simulink model "Inverse_Stewartplatform"  (R2024a)
settings: Solver=VariableStepAuto  StartTime=0.0  StopTime=0  RelTol=1e-3
settings Model: Creator=Challa  LastModifiedBy=Challa

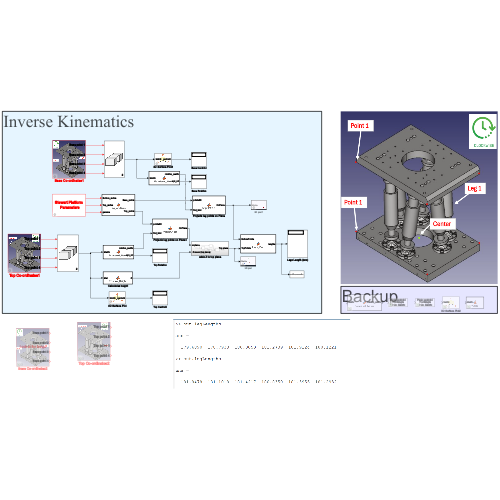
[thumbnail: Simulink's stored preview of the top-level diagram]
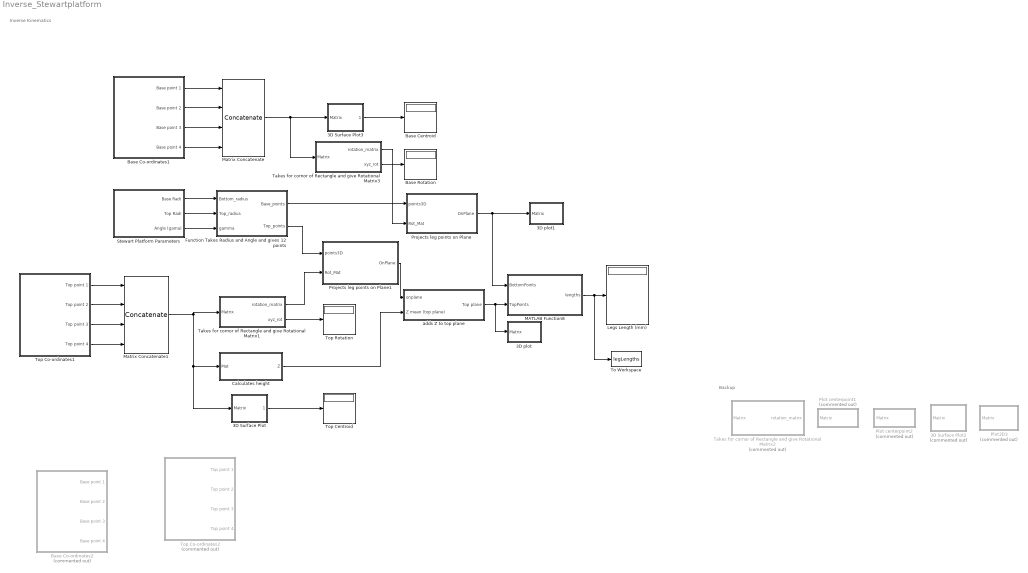
== system Inverse_Stewartplatform ==
  note: Backup
  note: Inverse Kinematics
  3D Surface Plot : Subsystem  mask(3D Surface Plot){color2='r'}
      mask prompts: color2 "color"
      mask help:
      | Input: 3xN matrix
      | output: 3D Surface Plot
      | Color: Changable by giving input
      | Finds Centerpoint and plots.
      mask Help:
      | Input: 3xN matrix
      | output: 3D Surface Plot
      | Color: Changable by giving input
      | Finds Centerpoint and plots.
      mask Display: image('XYZ2.png');
  3D Surface Plot2 : Subsystem  Commented=on  mask(3D Surface Plot){color2='b'}
      mask prompts: color2 "color"
      mask help:
      | Input: 3xN matrix
      | output: 3D Surface Plot
      | Color: Changable by giving input
      | Finds Centerpoint and plots.
      mask Help:
      | Input: 3xN matrix
      | output: 3D Surface Plot
      | Color: Changable by giving input
      | Finds Centerpoint and plots.
      mask Display: image('XYZ2.png');
  3D Surface Plot3 : Subsystem  mask(3D Surface Plot){color2='b'}
      mask prompts: color2 "color"
      mask help:
      | Input: 3xN matrix
      | output: 3D Surface Plot
      | Color: Changable by giving input
      | Finds Centerpoint and plots.
      mask Help:
      | Input: 3xN matrix
      | output: 3D Surface Plot
      | Color: Changable by giving input
      | Finds Centerpoint and plots.
      mask Display: image('XYZ2.png');
  3D plot : Subsystem  mask(3D Plot){color1='r'}
      mask prompts: color1 "color"
      mask help:
      | Input: 3xN matrix
      | output: 3D Plot
      | Color: Changable by giving input
      mask Help:
      | Input: 3xN matrix
      | output: 3D Plot
      | Color: Changable by giving input
      mask Display: image('XYZ.png');
  3D plot1 : Subsystem  mask(3D Plot){color1='b'}
      mask prompts: color1 "color"
      mask help:
      | Input: 3xN matrix
      | output: 3D Plot
      | Color: Changable by giving input
      mask Help:
      | Input: 3xN matrix
      | output: 3D Plot
      | Color: Changable by giving input
      mask Display: image('XYZ.png');
  Base Centroid : Display
  Base Co-ordinates1 : Subsystem  mask(Bottom / Base platform points){B1=[-82.47 112.5 -0.045], B2=[ 82.448 112.511 0.119], B3=[82.493 -112.496 0.045], B4=[-82.47 -112.514 -0.119]}
      mask prompts: B1 "Point 1 [X Y Z] (mm)"; B2 "Point 2 [X Y Z] (mm)"; B3 "Point 3 [X Y Z] (mm)"; B4 "Point 4 [X Y Z] (mm)"
      mask help:
      | Please look at diagram to give Bottom / Base platform points
      | Array [X Y Z] with respect to the Base platform Rectangle centre
      mask Help:
      | Please look at diagram to give Bottom / Base platform points
      | Array [X Y Z] with respect to the Base platform Rectangle centre
      mask Display:
      | disp('Look at the image');
      | image('Screenshot 2024-06-21 170647.png');
  Base Co-ordinates2 : Subsystem  Commented=on  mask(Bottom / Base platform points){B1=[-82.472,112.502,-0.038], B2=[ 82.45,112.512,0.108], B3=[82.493,-112.497,0.038], B4=[-82.472,-112.515,-0.108]}
      mask prompts: B1 "Point 1 [X Y Z] (mm)"; B2 "Point 2 [X Y Z] (mm)"; B3 "Point 3 [X Y Z] (mm)"; B4 "Point 4 [X Y Z] (mm)"
      mask help:
      | Please look at diagram to give Bottom / Base platform points
      | Array [X Y Z] with respect to the Base platform Rectangle centre
      mask Help:
      | Please look at diagram to give Bottom / Base platform points
      | Array [X Y Z] with respect to the Base platform Rectangle centre
      mask Display:
      | disp('Look at the image');
      | image('Screenshot 2024-06-21 170647.png');
  Base Rotation : Display
  Calculates height : MATLAB Function  TreatAsAtomicUnit=on
  Function Takes Radius and Angle and gives 12 points : MATLAB Function  TreatAsAtomicUnit=on
  Legs Length (mm) : Display
  MATLAB Function8 : MATLAB Function  TreatAsAtomicUnit=on
  Matrix Concatenate : Concatenate  NumInputs=4  Mode=Multidimensional array  ConcatenateDimension=2
  Matrix Concatenate1 : Concatenate  NumInputs=4  Mode=Multidimensional array  ConcatenateDimension=2
  Plot centerpoint1 : Subsystem  Commented=on
      mask Display: disp('Plots centroid \n Rectangle \n from Matrix');
  Plot centerpoint2 : Subsystem  Commented=on
      mask Display: disp('Plots centroid \n Rectangle \n from Matrix');
  Plot3D3 : MATLAB Function  Commented=on  TreatAsAtomicUnit=on
  Projects leg points on Plane : MATLAB Function  TreatAsAtomicUnit=on
  Projects leg points on Plane1 : MATLAB Function  TreatAsAtomicUnit=on
  Stewart Platform Parameters : Subsystem  mask(Gamma or Angle){B_R=130/2, T_R=125/2, Angle=20}
      mask prompts: B_R "Base Radius (mm)"; T_R "Top Radius(mm)"; Angle "Angle or Gama(deg)"
      mask help: Gamma is the half angle between 2 centres of leg
      mask Help: Gamma is the half angle between 2 centres of leg
      mask Display: disp('Stewart Platform \n Paramaters');
  Takes for cornor of Rectangle and give Rotational Matrix1 : MATLAB Function  TreatAsAtomicUnit=on
  Takes for cornor of Rectangle and give Rotational Matrix2 : MATLAB Function  Commented=on  TreatAsAtomicUnit=on
  Takes for cornor of Rectangle and give Rotational Matrix3 : MATLAB Function  TreatAsAtomicUnit=on
  To Workspace : ToWorkspace  VariableName=legLengths  SampleTime=-1
      settings: Save2DSignal=2-D array (concatenate along first dimension)
  Top Centroid : Display
  Top Co-ordinates1 : Subsystem  mask(Top / Moving Platform Points){T1=[-88.876 113.388 179.37], T2=[ 75.977 118.547 180.23], T3=[83.117 -106.291 180.494], T4=[-81.724 -111.522 179.634]}
      mask prompts: T1 "Point 1 [X Y Z] (mm)"; T2 "Point 2 [X Y Z] (mm)"; T3 "Point 3 [X Y Z] (mm)"; T4 "Point 4 [X Y Z] (mm)"
      mask help:
      | Please look at diagram to give Top / Moving Platform points
      | Array [X Y Z] with respect to the Base platform Rectangle centre
      mask Help:
      | Please look at diagram to give Top / Moving Platform points
      | Array [X Y Z] with respect to the Base platform Rectangle centre
      mask Display: image('Screenshot 2024-06-21 172342.png');
  Top Co-ordinates2 : Subsystem  Commented=on  mask(Top / Moving Platform Points){T1=[-83.58,104.326,181.88], T2=[ 81.26,109.403,180.886], T3=[88.251,-115.378,175.937], T4=[-76.569,-120.533,176.929]}
      mask prompts: T1 "Point 1 [X Y Z] (mm)"; T2 "Point 2 [X Y Z] (mm)"; T3 "Point 3 [X Y Z] (mm)"; T4 "Point 4 [X Y Z] (mm)"
      mask help:
      | Please look at diagram to give Top / Moving Platform points
      | Array [X Y Z] with respect to the Base platform Rectangle centre
      mask Help:
      | Please look at diagram to give Top / Moving Platform points
      | Array [X Y Z] with respect to the Base platform Rectangle centre
      mask Display: image('Screenshot 2024-06-21 172342.png');
  Top Rotation : Display
  adds Z to top plane : Subsystem
  wires:
  adds Z to top plane/1(Top plane) -> MATLAB Function8/2(TopPoints), 3D plot/1(Matrix)
  Top Co-ordinates1/4(Top point 4) -> Matrix Concatenate1/4
  Top Co-ordinates1/3(Top point 3) -> Matrix Concatenate1/3
  Takes for cornor of Rectangle and give Rotational Matrix3/2(xyz_rot) -> Base Rotation/1
  Top Co-ordinates1/2(Top point 2) -> Matrix Concatenate1/2
  Top Co-ordinates1/1(Top point 1) -> Matrix Concatenate1/1
  Base Co-ordinates1/1(Base point 1) -> Matrix Concatenate/1
  Stewart Platform Parameters/1(Base Radi) -> Function Takes Radius and Angle and gives 12 points/1(Bottom_radius)
  Base Co-ordinates1/4(Base point 4) -> Matrix Concatenate/4
  Stewart Platform Parameters/3(Angle (gama)) -> Function Takes Radius and Angle and gives 12 points/3(gamma)
  Base Co-ordinates1/3(Base point 3) -> Matrix Concatenate/3
  Base Co-ordinates1/2(Base point 2) -> Matrix Concatenate/2
  Projects leg points on Plane1/1(OnPlane) -> adds Z to top plane/1(onplane)
  Stewart Platform Parameters/2(Top Radi) -> Function Takes Radius and Angle and gives 12 points/2(Top_radius)
  Matrix Concatenate1/1 -> 3D Surface Plot/1(Matrix), Calculates height/1(Mat), Takes for cornor of Rectangle and give Rotational Matrix1/1(Matrix)
  Matrix Concatenate/1 -> 3D Surface Plot3/1(Matrix), Takes for cornor of Rectangle and give Rotational Matrix3/1(Matrix)
  Function Takes Radius and Angle and gives 12 points/1(Base_points) -> Projects leg points on Plane/1(points3D)
  Function Takes Radius and Angle and gives 12 points/2(Top_points) -> Projects leg points on Plane1/1(points3D)
  Takes for cornor of Rectangle and give Rotational Matrix1/1(rotation_matrix) -> Projects leg points on Plane1/2(Rot_Mat)
  Takes for cornor of Rectangle and give Rotational Matrix1/2(xyz_rot) -> Top Rotation/1
  Calculates height/1(Z) -> adds Z to top plane/2(" Z mean (top plane)")
  3D Surface Plot/1(centroid) -> Top Centroid/1
  3D Surface Plot3/1(centroid) -> Base Centroid/1
  Projects leg points on Plane/1(OnPlane) -> 3D plot1/1(Matrix), MATLAB Function8/1(BottomPoints)
  Takes for cornor of Rectangle and give Rotational Matrix3/1(rotation_matrix) -> Projects leg points on Plane/2(Rot_Mat)
  MATLAB Function8/1(lengths) -> To Workspace/1, Legs Length (mm)/1

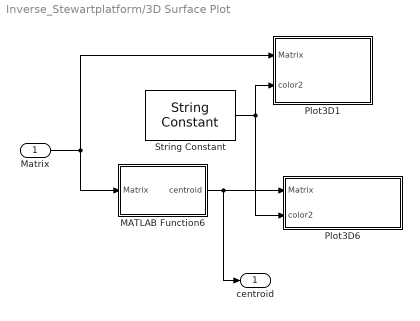
== system Inverse_Stewartplatform/3D Surface Plot ==
  Matrix : Inport
  MATLAB Function6 : MATLAB Function  TreatAsAtomicUnit=on
  Plot3D1 : MATLAB Function  TreatAsAtomicUnit=on
  Plot3D6 : MATLAB Function  TreatAsAtomicUnit=on
  String Constant : StringConstant  String=color2
  centroid : Outport
  wires:
  Matrix/1 -> Plot3D1/1(Matrix), MATLAB Function6/1(Matrix)
  MATLAB Function6/1(centroid) -> centroid/1, Plot3D6/1(Matrix)
  String Constant/1 -> Plot3D6/2(color2), Plot3D1/2(color2)

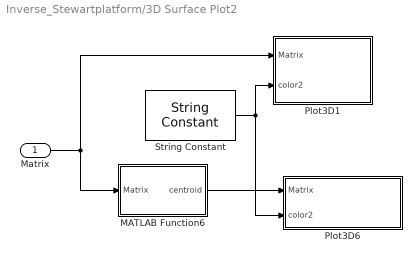
== system Inverse_Stewartplatform/3D Surface Plot2 ==
  Matrix : Inport
  MATLAB Function6 : MATLAB Function  TreatAsAtomicUnit=on
  Plot3D1 : MATLAB Function  TreatAsAtomicUnit=on
  Plot3D6 : MATLAB Function  TreatAsAtomicUnit=on
  String Constant : StringConstant  String=color2
  wires:
  Matrix/1 -> Plot3D1/1(Matrix), MATLAB Function6/1(Matrix)
  MATLAB Function6/1(centroid) -> Plot3D6/1(Matrix)
  String Constant/1 -> Plot3D6/2(color2), Plot3D1/2(color2)

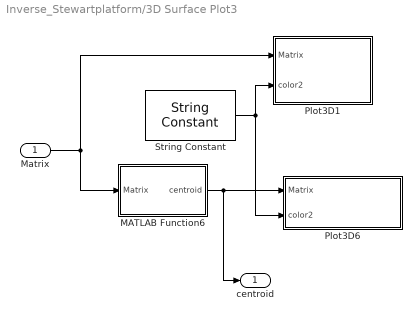
== system Inverse_Stewartplatform/3D Surface Plot3 ==
  Matrix : Inport
  MATLAB Function6 : MATLAB Function  TreatAsAtomicUnit=on
  Plot3D1 : MATLAB Function  TreatAsAtomicUnit=on
  Plot3D6 : MATLAB Function  TreatAsAtomicUnit=on
  String Constant : StringConstant  String=color2
  centroid : Outport
  wires:
  String Constant/1 -> Plot3D1/2(color2), Plot3D6/2(color2)
  MATLAB Function6/1(centroid) -> Plot3D6/1(Matrix), centroid/1
  Matrix/1 -> MATLAB Function6/1(Matrix), Plot3D1/1(Matrix)

== system Inverse_Stewartplatform/3D plot ==
  Matrix : Inport
  Plot3D1 : MATLAB Function  TreatAsAtomicUnit=on
  String Constant : StringConstant  String=color1
  wires:
  String Constant/1 -> Plot3D1/2(color1)
  Matrix/1 -> Plot3D1/1(Matrix)

== system Inverse_Stewartplatform/3D plot1 ==
  Matrix : Inport
  Plot3D1 : MATLAB Function  TreatAsAtomicUnit=on
  String Constant : StringConstant  String=color1
  wires:
  Matrix/1 -> Plot3D1/1(Matrix)
  String Constant/1 -> Plot3D1/2(color1)

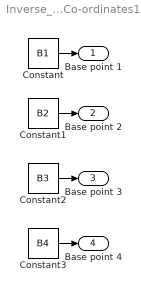
== system Inverse_Stewartplatform/Base Co-ordinates1 ==
  Constant : Constant  Value=B1
  Constant1 : Constant  Value=B2
  Constant2 : Constant  Value=B3
  Constant3 : Constant  Value=B4
  Base point 1 : Outport
  Base point 2 : Outport  Port=2
  Base point 3 : Outport  Port=3
  Base point 4 : Outport  Port=4
  wires:
  Constant/1 -> Base point 1/1
  Constant2/1 -> Base point 3/1
  Constant3/1 -> Base point 4/1
  Constant1/1 -> Base point 2/1

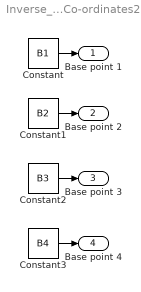
== system Inverse_Stewartplatform/Base Co-ordinates2 ==
  Constant : Constant  Value=B1
  Constant1 : Constant  Value=B2
  Constant2 : Constant  Value=B3
  Constant3 : Constant  Value=B4
  Base point 1 : Outport
  Base point 2 : Outport  Port=2
  Base point 3 : Outport  Port=3
  Base point 4 : Outport  Port=4
  wires:
  Constant/1 -> Base point 1/1
  Constant2/1 -> Base point 3/1
  Constant3/1 -> Base point 4/1
  Constant1/1 -> Base point 2/1

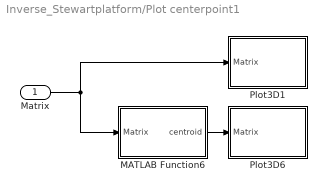
== system Inverse_Stewartplatform/Plot centerpoint1 ==
  Matrix : Inport
  MATLAB Function6 : MATLAB Function  TreatAsAtomicUnit=on
  Plot3D1 : MATLAB Function  TreatAsAtomicUnit=on
  Plot3D6 : MATLAB Function  TreatAsAtomicUnit=on
  wires:
  Matrix/1 -> Plot3D1/1(Matrix), MATLAB Function6/1(Matrix)
  MATLAB Function6/1(centroid) -> Plot3D6/1(Matrix)

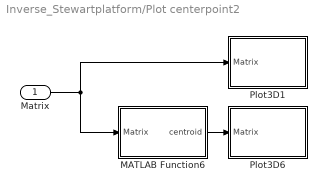
== system Inverse_Stewartplatform/Plot centerpoint2 ==
  Matrix : Inport
  MATLAB Function6 : MATLAB Function  TreatAsAtomicUnit=on
  Plot3D1 : MATLAB Function  TreatAsAtomicUnit=on
  Plot3D6 : MATLAB Function  TreatAsAtomicUnit=on
  wires:
  MATLAB Function6/1(centroid) -> Plot3D6/1(Matrix)
  Matrix/1 -> MATLAB Function6/1(Matrix), Plot3D1/1(Matrix)

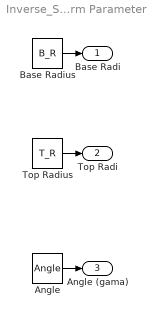
== system Inverse_Stewartplatform/Stewart Platform Parameters ==
  Angle : Constant  Value=Angle
  Base Radius : Constant  Value=B_R
  Top Radius : Constant  Value=T_R
  Base Radi : Outport
  Top Radi : Outport  Port=2
  Angle (gama) : Outport  Port=3
  wires:
  Angle/1 -> Angle (gama)/1
  Base Radius/1 -> Base Radi/1
  Top Radius/1 -> Top Radi/1

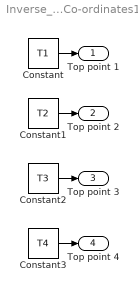
== system Inverse_Stewartplatform/Top Co-ordinates1 ==
  Constant : Constant  Value=T1
  Constant1 : Constant  Value=T2
  Constant2 : Constant  Value=T3
  Constant3 : Constant  Value=T4
  Top point 1 : Outport
  Top point 2 : Outport  Port=2
  Top point 3 : Outport  Port=3
  Top point 4 : Outport  Port=4
  wires:
  Constant/1 -> Top point 1/1
  Constant2/1 -> Top point 3/1
  Constant3/1 -> Top point 4/1
  Constant1/1 -> Top point 2/1

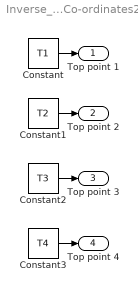
== system Inverse_Stewartplatform/Top Co-ordinates2 ==
  Constant : Constant  Value=T1
  Constant1 : Constant  Value=T2
  Constant2 : Constant  Value=T3
  Constant3 : Constant  Value=T4
  Top point 1 : Outport
  Top point 2 : Outport  Port=2
  Top point 3 : Outport  Port=3
  Top point 4 : Outport  Port=4
  wires:
  Constant/1 -> Top point 1/1
  Constant2/1 -> Top point 3/1
  Constant3/1 -> Top point 4/1
  Constant1/1 -> Top point 2/1

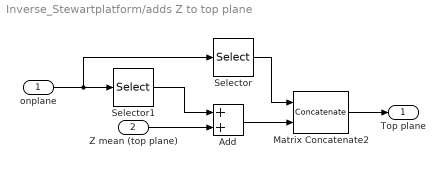
== system Inverse_Stewartplatform/adds Z to top plane ==
  onplane : Inport
  " Z mean (top plane)" : Inport  Port=2
  Add : Sum
  Matrix Concatenate2 : Concatenate  Mode=Multidimensional array
  Selector : Selector  NumberOfDimensions=2  InputPortWidth=3  IndexOptions=Index vector (dialog),Select all  Indices=[1 2],2  OutputSizes=1,1
  Selector1 : Selector  NumberOfDimensions=2  InputPortWidth=3  IndexOptions=Index vector (dialog),Select all  Indices=3,2  OutputSizes=1,1
  Top plane : Outport
  wires:
  onplane/1 -> Selector/1, Selector1/1
  Selector/1 -> Matrix Concatenate2/1
  Selector1/1 -> Add/1
  " Z mean (top plane)"/1 -> Add/2
  Add/1 -> Matrix Concatenate2/2
  Matrix Concatenate2/1 -> Top plane/1

== matlab function Inverse_Stewartplatform/Plot centerpoint2/Plot3D6 ==
  data: Matrix input
function Plot3D(Matrix)

figure(1)
x = Matrix(1, :);
y = Matrix(2, :);
z = Matrix(3, :);

% Create the 3D plot
plot3(x, y, z, 'o-', 'Color','r','LineWidth', 2);
xlabel('X Axis');
ylabel('Y Axis');
zlabel('Z Axis');


grid on


hold on;

% Connect the initial and final points
plot3([x(1) x(end)], [y(1) y(end)], [z(1) z(end)], 'o-', 'Color','r','LineWidth', 2);

hold on

end

== matlab function Inverse_Stewartplatform/Plot centerpoint1/Plot3D6 ==
  data: Matrix input
function Plot3D(Matrix)

figure(1)
x = Matrix(1, :);
y = Matrix(2, :);
z = Matrix(3, :);

% Create the 3D plot
plot3(x, y, z, 'o-', 'Color','b','LineWidth', 2);
xlabel('X Axis');
ylabel('Y Axis');
zlabel('Z Axis');


grid on


hold on;

% Connect the initial and final points
plot3([x(1) x(end)], [y(1) y(end)], [z(1) z(end)], 'o-', 'Color','b','LineWidth', 2);

hold on

end

== matlab function Inverse_Stewartplatform/Takes for cornor of Rectangle and give Rotational Matrix1 ==
  data: Matrix input; rotation_matrix output; xyz_rot output
function [rotation_matrix,xyz_rot] = Rotational_Matrix(Matrix)
    % A, B, C, D are the 3D coordinates of the rectangle's corners
    A = Matrix(:,1);
    B = Matrix(:,2);
    C = Matrix(:,3);
    D = Matrix(:,4);

    % Calculate the normal vector of the plane using cross product
    AB = B - A;
    AD = D - A;
    normal = cross(AB, AD);
    normal = normal / norm(normal); % Normalize the normal vector

    % Create orthogonal basis vectors on the plane
    e1 = AB / norm(AB); % First direction vector on the plane
    e2 = cross(normal, e1); % Second direction vector on the plane

    % Construct the rotation matrix from the plane's basis vectors
    rotation_matrix = [e1 e2 normal];

    % Calculate Euler angles (rotations in XYZ)
    % Assuming the rectangle is initially aligned with the XY plane,
    % we can calculate the rotations needed to align it with the given orientation.
    thetaX = atan2(normal(2), normal(3));
    thetaY = atan2(-normal(1), sqrt(normal(2)^2 + normal(3)^2));
    thetaZ = atan2(AB(2), AB(1));
    
    % Convert angles to degrees
    thetaX_deg = rad2deg(thetaX);
    thetaY_deg = rad2deg(thetaY);
    thetaZ_deg = rad2deg(thetaZ);

    xyz_rot = [thetaX_deg,thetaY_deg, thetaZ_deg];
end

== matlab function Inverse_Stewartplatform/Projects leg points on Plane1 ==
  data: points3D input; Rot_Mat input; OnPlane output
function OnPlane = ProjectOn3D( points3D, Rot_Mat )
    % Project points onto the XY plane in 3D
    
    % Perform the projection
    OnPlane = [Rot_Mat * points3D; zeros(1, size(points3D, 2))];
end

== matlab function Inverse_Stewartplatform/MATLAB Function8 ==
  data: BottomPoints input; TopPoints input; lengths output
function lengths = Legs_Plot( BottomPoints, TopPoints)

    % Plotting legs
    figure(1)
    count = 0;
    while count < 6
        count = count + 1;  % Increment the counter
        i = count;
        % Create the 3D plot
        plot3([TopPoints(1,i) BottomPoints(1,i)], [TopPoints(2,i) BottomPoints(2,i)], [TopPoints(3,i) BottomPoints(3,i)], 'Color','g','LineWidth', 2);
        hold on
    end
lengths = [0 0 0 0 0 0];
count = 0;
    while count < 6
        count = count + 1;  % Increment the counter
        i = count;
        % Create the 3D plot
        d = sqrt((TopPoints(1,i) - BottomPoints(1,i))^2 + (TopPoints(2,i)-BottomPoints(2,i))^2 + (TopPoints(3,i) - BottomPoints(3,i))^2);
        lengths(i) = d;
    end
end

== matlab function Inverse_Stewartplatform/Calculates height ==
  data: Mat input; Z output
function Z = Topplate_Height(Mat)

Z = mean(Mat(3,:));


% centroid = mean(Mat, 2);
% Z = sqrt(sum((centroid - [0 0 0]).^2));


% check if the height from bottom surface  or form bottom centre point

== matlab function Inverse_Stewartplatform/3D Surface Plot/Plot3D6 ==
  data: Matrix input; color2 input
function Plot3D(Matrix,color2)

figure(1)
x = Matrix(1, :);
y = Matrix(2, :);
z = Matrix(3, :);

% Create the 3D plot
plot3(x, y, z, 'o-', 'Color',color2,'LineWidth', 2);
xlabel('X Axis');
ylabel('Y Axis');
zlabel('Z Axis');


grid on


hold on;

% Connect the initial and final points
plot3([x(1) x(end)], [y(1) y(end)], [z(1) z(end)], 'o-', 'Color',color2,'LineWidth', 2);

hold on

end

== matlab function Inverse_Stewartplatform/Takes for cornor of Rectangle and give Rotational Matrix2 ==
  data: Matrix input; rotation_matrix output
function rotation_matrix  = Rotational_Matrix(Matrix)
    % A, B, C, D are the 3D coordinates of the rectangle's corners
    A = Matrix(:,1);
    B = Matrix(:,2);
    C = Matrix(:,3);
    D = Matrix(:,4);

    % Calculate the normal vector of the plane using cross product
    AB = B - A;
    AD = D - A;
    normal = cross(AB, AD);
    normal = normal / norm(normal); % Normalize the normal vector

    % Create orthogonal basis vectors on the plane
    e1 = AB / norm(AB); % First direction vector on the plane
    e2 = cross(normal, e1); % Second direction vector on the plane

    % Construct the rotation matrix from the plane's basis vectors
    rotation_matrix = [e1 e2 normal];
   
end

== matlab function Inverse_Stewartplatform/Takes for cornor of Rectangle and give Rotational Matrix3 ==
  data: Matrix input; rotation_matrix output; xyz_rot output
function [rotation_matrix,xyz_rot] = Rotational_Matrix(Matrix)
    % A, B, C, D are the 3D coordinates of the rectangle's corners
    A = Matrix(:,1);
    B = Matrix(:,2);
    C = Matrix(:,3);
    D = Matrix(:,4);

    % Calculate the normal vector of the plane using cross product
    AB = B - A;
    AD = D - A;
    normal = cross(AB, AD);
    normal = normal / norm(normal); % Normalize the normal vector

    % Create orthogonal basis vectors on the plane
    e1 = AB / norm(AB); % First direction vector on the plane
    e2 = cross(normal, e1); % Second direction vector on the plane

    % Construct the rotation matrix from the plane's basis vectors
    rotation_matrix = [e1 e2 normal];

    % Calculate Euler angles (rotations in XYZ)
    % Assuming the rectangle is initially aligned with the XY plane,
    % we can calculate the rotations needed to align it with the given orientation.
    thetaX = atan2(normal(2), normal(3));
    thetaY = atan2(-normal(1), sqrt(normal(2)^2 + normal(3)^2));
    thetaZ = atan2(AB(2), AB(1));
    
    % Convert angles to degrees
    thetaX_deg = rad2deg(thetaX);
    thetaY_deg = rad2deg(thetaY);
    thetaZ_deg = rad2deg(thetaZ);

    xyz_rot = [thetaX_deg,thetaY_deg, thetaZ_deg];
end

== matlab function Inverse_Stewartplatform/Plot3D3 ==
  data: Matrix input
function Plot3D(Matrix)

figure(1)
x = Matrix(1, :);
y = Matrix(2, :);
z = Matrix(3, :);

% Create the 3D plot
plot3(x, y, z, 'o-', 'Color','b','LineWidth', 2);
xlabel('X Axis');
ylabel('Y Axis');
zlabel('Z Axis');

axis equal
grid on


hold on;

% Connect the initial and final points
plot3([x(1) x(end)], [y(1) y(end)], [z(1) z(end)], 'o-', 'Color','b','LineWidth', 2);

hold on

end

== matlab function Inverse_Stewartplatform/Function Takes Radius and Angle and gives 12 points ==
  data: Bottom_radius input; Base_points output; Top_radius input; gamma input; Top_points output
function [Base_points, Top_points]= Leg_locations(Bottom_radius, Top_radius, gamma)
    % Define the fixed and moving platform geometry (attachment points)
    % Fixed platform attachment points (in the base frame)
    r1 = Bottom_radius;
    r2 = Top_radius;
    A0=[r1*cosd(60-gamma) r1*sind(60-gamma) 0]'; 
    B0=[r1*cosd(60+gamma) r1*sind(60+gamma) 0]'; 
    C0=[-r1*cosd(gamma) r1*sind(gamma) 0]'; 
    D0=[-r1*cosd(gamma) -r1*sind(gamma) 0]'; 
    E0=[r1*cosd(60+gamma) -r1*sind(60+gamma) 0]'; 
    F0=[r1*cosd(60-gamma) -r1*sind(60-gamma) 0]'; 
    
    B = [A0 B0 C0 D0 E0 F0];
    
    % Moving platform attachment points (in the moving frame)
    
    A1=[r2*cosd(gamma) r2*sind(gamma) 0]';
    B1=[-r2*sind(30-gamma) r2*cosd(30-gamma) 0]';
    C1=[-r2*sind(30+gamma) r2*cosd(30+gamma) 0]';
    D1=[-r2*sind(30+gamma) -r2*cosd(30+gamma) 0]';
    E1=[-r2*sind(30-gamma) -r2*cosd(30-gamma) 0]';
    F1=[r2*cosd(gamma) -r2*sind(gamma) 0]';
    
    P = [A1 B1 C1 D1 E1 F1];
    
Base_points  = B;
Top_points = P;

== matlab function Inverse_Stewartplatform/3D Surface Plot2/Plot3D6 ==
  data: Matrix input; color2 input
function Plot3D(Matrix,color2)

figure(1)
x = Matrix(1, :);
y = Matrix(2, :);
z = Matrix(3, :);

% Create the 3D plot
plot3(x, y, z, 'o-', 'Color',color2,'LineWidth', 2);
xlabel('X Axis');
ylabel('Y Axis');
zlabel('Z Axis');


grid on


hold on;

% Connect the initial and final points
plot3([x(1) x(end)], [y(1) y(end)], [z(1) z(end)], 'o-', 'Color',color2,'LineWidth', 2);

hold on

end

== matlab function Inverse_Stewartplatform/3D Surface Plot3/MATLAB Function6 ==
  data: Matrix input; centroid output
function centroid  = FindCentroid(Matrix)
    % This function calculates the centroid of a 3xN matrix
    % points: a 3xN matrix where each column represents a point in 3D space
    % centroid: a 3x1 vector representing the center point of the given points

    % Validate input
    if size(Matrix, 1) ~= 3
        error('Input matrix must have 3 rows');
    end

    % Calculate the centroid
    centroid = mean(Matrix, 2);
end

== matlab function Inverse_Stewartplatform/3D Surface Plot3/Plot3D1 ==
  data: Matrix input; color2 input
function Plot3D(Matrix, color2)

figure(1)
x = Matrix(1, :);
y = Matrix(2, :);
z = Matrix(3, :);

% Create the 3D plot
plot3(x, y, z, 'o-', 'Color',color2,'LineWidth', 2);
hold on
fill3(x, y, z, color2, 'FaceAlpha', 0.2)
xlabel('X Axis');
ylabel('Y Axis');
zlabel('Z Axis');

axis equal
grid on


hold on;

% Connect the initial and final points
plot3([x(1) x(end)], [y(1) y(end)], [z(1) z(end)], 'o-', 'Color',color2,'LineWidth', 2);

hold on

end

== matlab function Inverse_Stewartplatform/3D Surface Plot3/Plot3D6 ==
  data: Matrix input; color2 input
function Plot3D(Matrix,color2)

figure(1)
x = Matrix(1, :);
y = Matrix(2, :);
z = Matrix(3, :);

% Create the 3D plot
plot3(x, y, z, 'o-', 'Color',color2,'LineWidth', 2);
xlabel('X Axis');
ylabel('Y Axis');
zlabel('Z Axis');


grid on


hold on;

% Connect the initial and final points
plot3([x(1) x(end)], [y(1) y(end)], [z(1) z(end)], 'o-', 'Color',color2,'LineWidth', 2);

hold on

end

== matlab function Inverse_Stewartplatform/3D plot/Plot3D1 ==
  data: Matrix input; color1 input
function Plot3D(Matrix,color1)

figure(1)
x = Matrix(1, :);
y = Matrix(2, :);
z = Matrix(3, :);

% Create the 3D plot
plot3(x, y, z, 'o-', 'color',color1,'LineWidth', 2);
xlabel('X Axis');
ylabel('Y Axis');
zlabel('Z Axis');

axis equal
grid on


hold on;

% Connect the initial and final points
plot3([x(1) x(end)], [y(1) y(end)], [z(1) z(end)], 'o-', 'Color',color1,'LineWidth', 2);

hold on

end

== matlab function Inverse_Stewartplatform/3D plot1/Plot3D1 ==
  data: Matrix input; color1 input
function Plot3D(Matrix,color1)

figure(1)
x = Matrix(1, :);
y = Matrix(2, :);
z = Matrix(3, :);

% Create the 3D plot
plot3(x, y, z, 'o-', 'color',color1,'LineWidth', 2);
xlabel('X Axis');
ylabel('Y Axis');
zlabel('Z Axis');

axis equal
grid on


hold on;

% Connect the initial and final points
plot3([x(1) x(end)], [y(1) y(end)], [z(1) z(end)], 'o-', 'Color',color1,'LineWidth', 2);

hold on

end

== matlab function Inverse_Stewartplatform/3D Surface Plot2/MATLAB Function6 ==
  data: Matrix input; centroid output
function centroid  = FindCentroid(Matrix)
    % This function calculates the centroid of a 3xN matrix
    % points: a 3xN matrix where each column represents a point in 3D space
    % centroid: a 3x1 vector representing the center point of the given points

    % Validate input
    if size(Matrix, 1) ~= 3
        error('Input matrix must have 3 rows');
    end

    % Calculate the centroid
    centroid = mean(Matrix, 2);
end

== matlab function Inverse_Stewartplatform/3D Surface Plot2/Plot3D1 ==
  data: Matrix input; color2 input
function Plot3D(Matrix, color2)

figure(1)
x = Matrix(1, :);
y = Matrix(2, :);
z = Matrix(3, :);

% Create the 3D plot
plot3(x, y, z, 'o-', 'Color',color2,'LineWidth', 2);
hold on
fill3(x, y, z, color2, 'FaceAlpha', 0.2)
xlabel('X Axis');
ylabel('Y Axis');
zlabel('Z Axis');

axis equal
grid on


hold on;

% Connect the initial and final points
plot3([x(1) x(end)], [y(1) y(end)], [z(1) z(end)], 'o-', 'Color',color2,'LineWidth', 2);

hold on

end

== matlab function Inverse_Stewartplatform/Plot centerpoint2/MATLAB Function6 ==
  data: Matrix input; centroid output
function centroid  = FindCentroid(Matrix)
    % This function calculates the centroid of a 3xN matrix
    % points: a 3xN matrix where each column represents a point in 3D space
    % centroid: a 3x1 vector representing the center point of the given points

    % Validate input
    if size(Matrix, 1) ~= 3
        error('Input matrix must have 3 rows');
    end

    % Calculate the centroid
    centroid = mean(Matrix, 2);
end

== matlab function Inverse_Stewartplatform/3D Surface Plot/MATLAB Function6 ==
  data: Matrix input; centroid output
function centroid  = FindCentroid(Matrix)
    % This function calculates the centroid of a 3xN matrix
    % points: a 3xN matrix where each column represents a point in 3D space
    % centroid: a 3x1 vector representing the center point of the given points

    % Validate input
    if size(Matrix, 1) ~= 3
        error('Input matrix must have 3 rows');
    end

    % Calculate the centroid
    centroid = mean(Matrix, 2);
end

== matlab function Inverse_Stewartplatform/3D Surface Plot/Plot3D1 ==
  data: Matrix input; color2 input
function Plot3D(Matrix, color2)

figure(1)
x = Matrix(1, :);
y = Matrix(2, :);
z = Matrix(3, :);

% Create the 3D plot
plot3(x, y, z, 'o-', 'Color',color2,'LineWidth', 2);
hold on
fill3(x, y, z, color2, 'FaceAlpha', 0.2)
xlabel('X Axis');
ylabel('Y Axis');
zlabel('Z Axis');

axis equal
grid on


hold on;

% Connect the initial and final points
plot3([x(1) x(end)], [y(1) y(end)], [z(1) z(end)], 'o-', 'Color',color2,'LineWidth', 2);

hold on

end

== matlab function Inverse_Stewartplatform/Projects leg points on Plane ==
  data: points3D input; Rot_Mat input; OnPlane output
function OnPlane = ProjectOn3D( points3D, Rot_Mat )
    % Project points onto the XY plane in 3D
    
    % Perform the projection
    OnPlane = [Rot_Mat * points3D; zeros(1, size(points3D, 2))];
end

== matlab function Inverse_Stewartplatform/Plot centerpoint1/MATLAB Function6 ==
  data: Matrix input; centroid output
function centroid  = FindCentroid(Matrix)
    % This function calculates the centroid of a 3xN matrix
    % points: a 3xN matrix where each column represents a point in 3D space
    % centroid: a 3x1 vector representing the center point of the given points

    % Validate input
    if size(Matrix, 1) ~= 3
        error('Input matrix must have 3 rows');
    end

    % Calculate the centroid
    centroid = mean(Matrix, 2);
end

== matlab function Inverse_Stewartplatform/Plot centerpoint1/Plot3D1 ==
  data: Matrix input
function Plot3D(Matrix)

figure(1)
x = Matrix(1, :);
y = Matrix(2, :);
z = Matrix(3, :);

% Create the 3D plot
plot3(x, y, z, 'o-', 'Color','b','LineWidth', 2);
hold on
fill3(x, y, z, 'b', 'FaceAlpha', 0.2)
xlabel('X Axis');
ylabel('Y Axis');
zlabel('Z Axis');

axis equal
grid on


hold on;

% Connect the initial and final points
plot3([x(1) x(end)], [y(1) y(end)], [z(1) z(end)], 'o-', 'Color','b','LineWidth', 2);

hold on

end

== matlab function Inverse_Stewartplatform/Plot centerpoint2/Plot3D1 ==
  data: Matrix input
function Plot3D(Matrix)

figure(1)
x = Matrix(1, :);
y = Matrix(2, :);
z = Matrix(3, :);

% Create the 3D plot
plot3(x, y, z, 'o-', 'Color','r','LineWidth', 2);
hold on
fill3(x, y, z, 'r', 'FaceAlpha', 0.2)
xlabel('X Axis');
ylabel('Y Axis');
zlabel('Z Axis');

axis equal
grid on


hold on;

% Connect the initial and final points
plot3([x(1) x(end)], [y(1) y(end)], [z(1) z(end)], 'o-', 'Color','r','LineWidth', 2);

hold on

end
